simulink model "distributed"  (R2022a)
settings: Solver=VariableStepAuto  StartTime=0.0  StopTime=T_fin  FixedStep=0.0025  RelTol=1e-3
values from neighbouring files (symbols this model uses):
  A = A-B*k_leader    [project.m]
  Ad = [0 0 1 0 0 0; 1 0 0 0 0 0;0 1 0 0 0 0; 1 0 0 0 0 0; 0 0 0 0 0 0; 0 0 1 0 0 0]    [project.m]
  B = [0; -9.9453]    [project.m]
  C = [708.27 0]    [project.m]
  c = 5    [project.m]
  D_ = zeros(2,1)'    [project.m]
  F = P2*C'*inv(R)    [project.m]
  G = diag([1 0 0 0 1 0])    [project.m]
  K = inv(R)*B'*P    [project.m]
  L_leader = acker(A',C',[-1,-2])'    [project.m]
  X0 = [1/C(1) 1/800]'    [project.m]
settings Model: Creator=Giacomo  LastModifiedBy=Utente
settings DataIOCC: ReturnWorkspaceOutputs=off

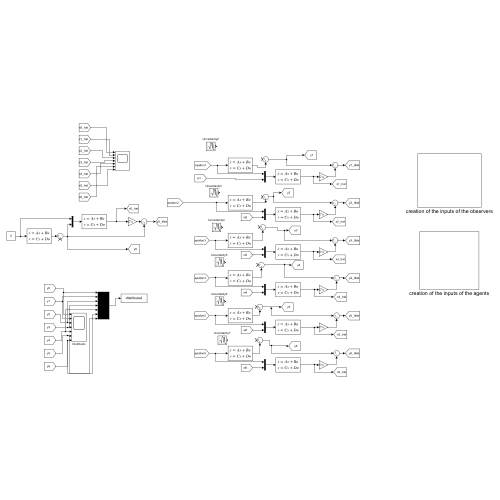
[thumbnail: Simulink's stored preview of the top-level diagram]
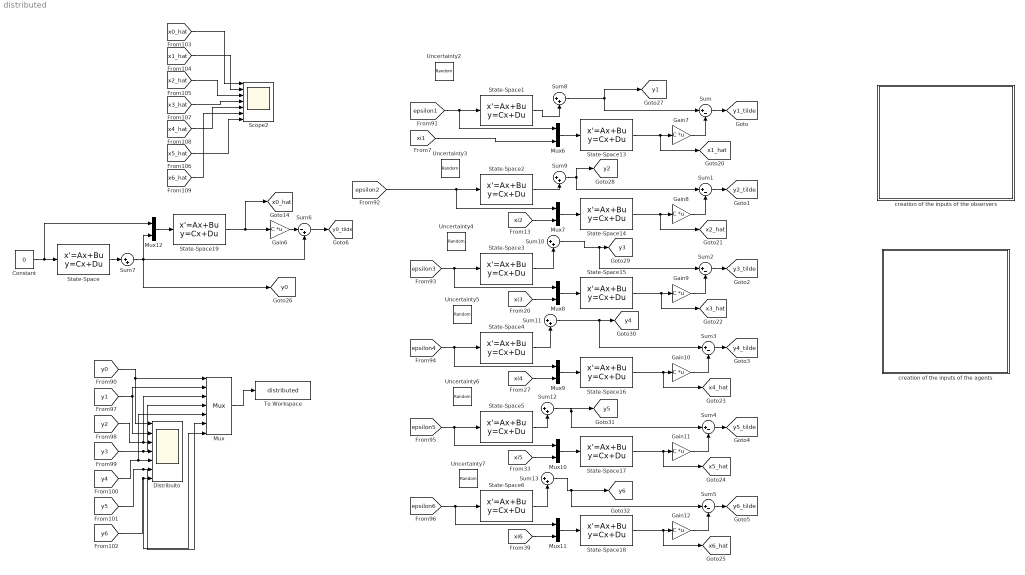
== system distributed ==
  Constant : Constant  Value=0
  Distribuito : Scope  NumInputPorts=7
  Gain{6..12} (7 alike) : Gain  Gain=C  Multiplication=Matrix(K*u)
  Mux : Mux  Inputs=7
  Mux{6..12} (7 alike) : Mux  Inputs=2
  Scope2 : Scope  NumInputPorts=7
  State-Space : StateSpace  A=A  B=B  C=C  D=0  InitialCondition=X0
  State-Space1 : StateSpace  A=A  B=B*c*K  C=C  D=D_  InitialCondition=[2/C(1) 1/800]'
  State-Space{13..18} (6 alike) : StateSpace  A=A  B=[B*c*K -c*F]  C=eye(2)  D=zeros(2,3)  InitialCondition=zeros(1,2)
  State-Space19 : StateSpace  A=A - L_leader*C  B=[B L_leader]  C=eye(2)  D=zeros(2,2)  InitialCondition=zeros(1,2)
  State-Space2 : StateSpace  A=A  B=B*c*K  C=C  D=D_  InitialCondition=[0 2/800]'
  State-Space3 : StateSpace  A=A  B=B*c*K  C=C  D=D_  InitialCondition=[-1/C(1) -1/800]
  State-Space4 : StateSpace  A=A  B=B*c*K  C=C  D=D_  InitialCondition=[3/C(1) -3/800]'
  State-Space5 : StateSpace  A=A  B=B*c*K  C=C  D=D_  InitialCondition=[2/C(1) 4/800]'
  State-Space6 : StateSpace  A=A  B=B*c*K  C=C  D=D_  InitialCondition=[-2/C(1) 0]'
  Sum{,1..5} (6 alike) : Sum  Inputs=|+-
  Sum{7..13} (7 alike) : Sum  Inputs=|++
  Sum6 : Sum  Inputs=|-+
  To Workspace : ToWorkspace  VariableName=distributed  SaveFormat=Timeseries  SampleTime=-1
  Uncertainty2 : RandomNumber  Mean=zeros(1,1)  Seed=2  SampleTime=0.2
  Uncertainty3 : RandomNumber  Mean=zeros(1,1)  Variance=0.5  Seed=7  SampleTime=0.1
  Uncertainty4 : RandomNumber  Mean=zeros(1,1)  Variance=0.2  Seed=7  SampleTime=0.1
  Uncertainty5 : RandomNumber  Mean=zeros(1,1)  Variance=0.7  Seed=3  SampleTime=0.1
  Uncertainty6 : RandomNumber  Mean=zeros(1,1)  Variance=0.1  Seed=1  SampleTime=0.1
  Uncertainty7 : RandomNumber  Mean=zeros(1,1)  Variance=0.4  Seed=3  SampleTime=0.1
  creation of the inputs of the agents : Subsystem
  creation of the inputs of the observers : Subsystem
  tag scope: x0_hat=global, x1_hat=global, x2_hat=global, x3_hat=global, x4_hat=global, x5_hat=global, x6_hat=global, y0=global, y0_tilde=global, y1=global, y1_tilde=global, y2=global, y2_tilde=global, y3=global, y3_tilde=global, y4=global, y4_tilde=global, y5=global, y5_tilde=global, y6=global, y6_tilde=global
  wires:
  Gain7/1 -> Sum/2
  Sum2/1 -> [y3_tilde]
  [xi2] -> Mux7/2
  [xi6] -> Mux11/2
  Mux8/1 -> State-Space15/1
  [xi3] -> Mux8/2
  [xi4] -> Mux9/2
  [xi5] -> Mux10/2
  [epsilon3] -> Mux8/1, State-Space3/1
  Mux6/1 -> State-Space13/1
  [epsilon6] -> State-Space6/1, Mux11/1
  [epsilon1] -> Mux6/1, State-Space1/1
  [epsilon5] -> State-Space5/1, Mux10/1
  Mux12/1 -> State-Space19/1
  Sum4/1 -> [y5_tilde]
  Mux9/1 -> State-Space16/1
  Sum5/1 -> [y6_tilde]
  Sum1/1 -> [y2_tilde]
  Gain12/1 -> Sum5/2
  [xi1] -> Mux6/2
  State-Space14/1 -> [x2_hat], Gain8/1
  [epsilon2] -> State-Space2/1, Mux7/1
  State-Space13/1 -> Gain7/1, [x1_hat]
  State-Space17/1 -> [x5_hat], Gain11/1
  Sum/1 -> [y1_tilde]
  Sum3/1 -> [y4_tilde]
  Gain11/1 -> Sum4/2
  State-Space19/1 -> Gain6/1, [x0_hat]
  [epsilon4] -> State-Space4/1, Mux9/1
  State-Space18/1 -> [x6_hat], Gain12/1
  State-Space15/1 -> [x3_hat], Gain9/1
  Gain8/1 -> Sum1/2
  Mux11/1 -> State-Space18/1
  Gain10/1 -> Sum3/2
  Sum6/1 -> [y0_tilde]
  State-Space16/1 -> [x4_hat], Gain10/1
  Gain9/1 -> Sum2/2
  Mux10/1 -> State-Space17/1
  Constant/1 -> Mux12/1, State-Space/1
  [y6] -> Mux/7, Distribuito/7
  [y5] -> Mux/6, Distribuito/6
  [y4] -> Distribuito/5, Mux/5
  [y3] -> Mux/4, Distribuito/4
  [y2] -> Mux/3, Distribuito/3
  [y1] -> Mux/2, Distribuito/2
  [y0] -> Mux/1, Distribuito/1
  Gain6/1 -> Sum6/1
  State-Space/1 -> Sum7/1
  Sum7/1 -> Mux12/2, Sum6/2, [y0]
  State-Space1/1 -> Sum8/2
  Sum8/1 -> [y1], Sum/1
  State-Space2/1 -> Sum9/2
  Sum9/1 -> Sum1/1, [y2]
  State-Space3/1 -> Sum10/2
  Sum10/1 -> Sum2/1, [y3]
  State-Space4/1 -> Sum11/2
  Sum11/1 -> Sum3/1, [y4]
  State-Space5/1 -> Sum12/2
  Sum12/1 -> Sum4/1, [y5]
  State-Space6/1 -> Sum13/2
  Sum13/1 -> Sum5/1, [y6]
  Mux/1 -> To Workspace/1
  [x0_hat] -> Scope2/1
  [x6_hat] -> Scope2/6
  [x3_hat] -> Scope2/4
  [x1_hat] -> Scope2/2
  [x2_hat] -> Scope2/3
  [x4_hat] -> Scope2/5
  [x5_hat] -> Scope2/7
  Mux7/1 -> State-Space14/1

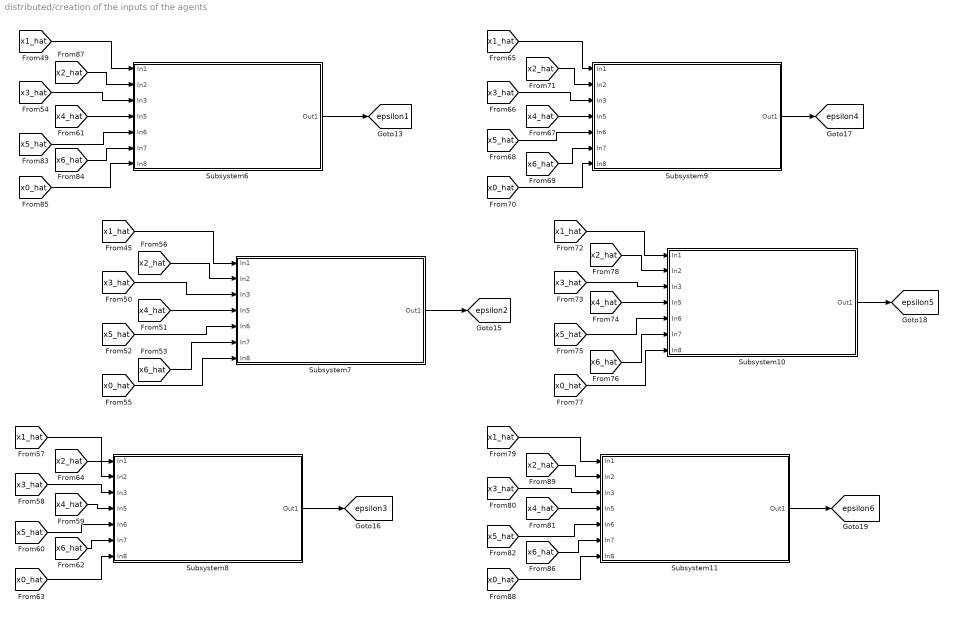
== system distributed/creation of the inputs of the agents ==
  Subsystem10 : Subsystem
  Subsystem11 : Subsystem
  Subsystem6 : Subsystem
  Subsystem7 : Subsystem
  Subsystem8 : Subsystem
  Subsystem9 : Subsystem
  tag scope: epsilon1=global, epsilon2=global, epsilon3=global, epsilon4=global, epsilon5=global, epsilon6=global
  wires:
  [x2_hat] -> Subsystem11/2(In2)
  Subsystem7/1(Out1) -> [epsilon2]
  [x1_hat] -> Subsystem10/1(In1)
  [x6_hat] -> Subsystem6/6(In7)
  [x3_hat] -> Subsystem8/3(In3)
  [x3_hat] -> Subsystem11/3(In3)
  [x5_hat] -> Subsystem6/5(In6)
  [x6_hat] -> Subsystem11/6(In7)
  [x4_hat] -> Subsystem6/4(In5)
  [x0_hat] -> Subsystem7/7(In8)
  [x1_hat] -> Subsystem9/1(In1)
  [x5_hat] -> Subsystem11/5(In6)
  Subsystem11/1(Out1) -> [epsilon6]
  [x3_hat] -> Subsystem10/3(In3)
  [x4_hat] -> Subsystem8/4(In5)
  Subsystem10/1(Out1) -> [epsilon5]
  [x3_hat] -> Subsystem7/3(In3)
  [x3_hat] -> Subsystem9/3(In3)
  Subsystem9/1(Out1) -> [epsilon4]
  [x0_hat] -> Subsystem10/7(In8)
  [x1_hat] -> Subsystem8/1(In1)
  [x6_hat] -> Subsystem7/6(In7)
  [x0_hat] -> Subsystem8/7(In8)
  [x5_hat] -> Subsystem10/5(In6)
  [x6_hat] -> Subsystem10/6(In7)
  [x5_hat] -> Subsystem7/5(In6)
  [x2_hat] -> Subsystem10/2(In2)
  [x4_hat] -> Subsystem7/4(In5)
  [x0_hat] -> Subsystem9/7(In8)
  [x4_hat] -> Subsystem9/4(In5)
  [x2_hat] -> Subsystem9/2(In2)
  Subsystem8/1(Out1) -> [epsilon3]
  [x5_hat] -> Subsystem8/5(In6)
  [x5_hat] -> Subsystem9/5(In6)
  [x4_hat] -> Subsystem10/4(In5)
  [x4_hat] -> Subsystem11/4(In5)
  [x1_hat] -> Subsystem7/1(In1)
  [x3_hat] -> Subsystem6/3(In3)
  [x0_hat] -> Subsystem11/7(In8)
  [x2_hat] -> Subsystem7/2(In2)
  Subsystem6/1(Out1) -> [epsilon1]
  [x0_hat] -> Subsystem6/7(In8)
  [x1_hat] -> Subsystem11/1(In1)
  [x2_hat] -> Subsystem8/2(In2)
  [x6_hat] -> Subsystem9/6(In7)
  [x2_hat] -> Subsystem6/2(In2)
  [x1_hat] -> Subsystem6/1(In1)
  [x6_hat] -> Subsystem8/6(In7)

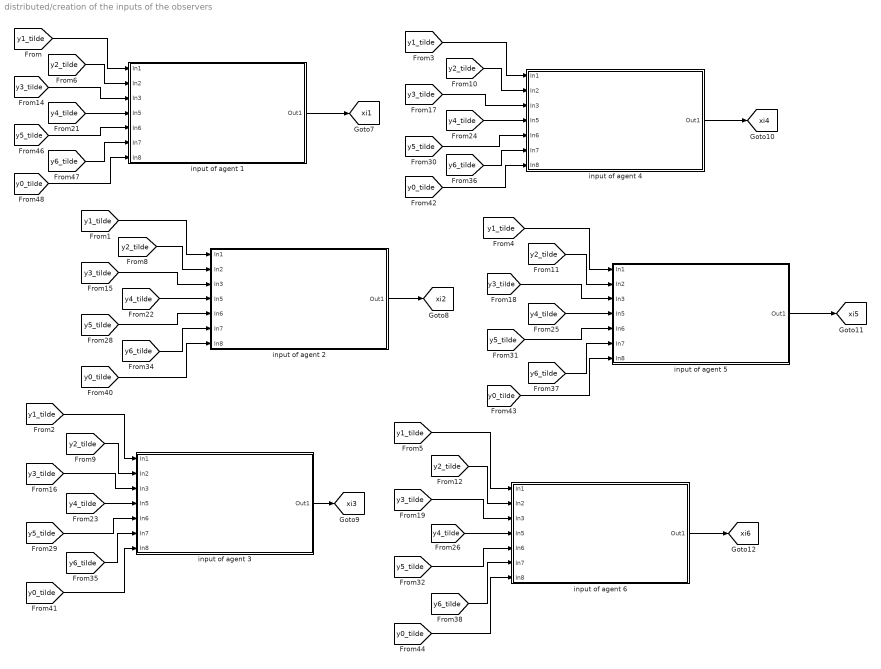
== system distributed/creation of the inputs of the observers ==
  input of agent 1 : Subsystem
  input of agent 2 : Subsystem
  input of agent 3 : Subsystem
  input of agent 4 : Subsystem
  input of agent 5 : Subsystem
  input of agent 6 : Subsystem
  tag scope: xi1=global, xi2=global, xi3=global, xi4=global, xi5=global, xi6=global
  wires:
  [y6_tilde] -> input of agent 5/6(In7)
  [y2_tilde] -> input of agent 2/2(In2)
  [y5_tilde] -> input of agent 3/5(In6)
  [y2_tilde] -> input of agent 5/2(In2)
  [y0_tilde] -> input of agent 1/7(In8)
  [y5_tilde] -> input of agent 4/5(In6)
  [y6_tilde] -> input of agent 4/6(In7)
  [y0_tilde] -> input of agent 6/7(In8)
  [y5_tilde] -> input of agent 1/5(In6)
  input of agent 3/1(Out1) -> [xi3]
  [y1_tilde] -> input of agent 3/1(In1)
  [y0_tilde] -> input of agent 3/7(In8)
  [y1_tilde] -> input of agent 2/1(In1)
  [y5_tilde] -> input of agent 5/5(In6)
  input of agent 6/1(Out1) -> [xi6]
  [y6_tilde] -> input of agent 3/6(In7)
  [y4_tilde] -> input of agent 4/4(In5)
  [y3_tilde] -> input of agent 4/3(In3)
  [y6_tilde] -> input of agent 1/6(In7)
  [y1_tilde] -> input of agent 1/1(In1)
  [y4_tilde] -> input of agent 1/4(In5)
  [y2_tilde] -> input of agent 6/2(In2)
  [y2_tilde] -> input of agent 4/2(In2)
  [y3_tilde] -> input of agent 3/3(In3)
  [y5_tilde] -> input of agent 6/5(In6)
  [y6_tilde] -> input of agent 2/6(In7)
  [y4_tilde] -> input of agent 5/4(In5)
  [y3_tilde] -> input of agent 5/3(In3)
  [y4_tilde] -> input of agent 6/4(In5)
  [y0_tilde] -> input of agent 4/7(In8)
  [y0_tilde] -> input of agent 5/7(In8)
  [y1_tilde] -> input of agent 6/1(In1)
  [y4_tilde] -> input of agent 2/4(In5)
  input of agent 1/1(Out1) -> [xi1]
  [y3_tilde] -> input of agent 6/3(In3)
  [y3_tilde] -> input of agent 1/3(In3)
  [y6_tilde] -> input of agent 6/6(In7)
  [y1_tilde] -> input of agent 4/1(In1)
  [y3_tilde] -> input of agent 2/3(In3)
  [y4_tilde] -> input of agent 3/4(In5)
  [y2_tilde] -> input of agent 3/2(In2)
  [y0_tilde] -> input of agent 2/7(In8)
  input of agent 4/1(Out1) -> [xi4]
  input of agent 2/1(Out1) -> [xi2]
  [y5_tilde] -> input of agent 2/5(In6)
  [y1_tilde] -> input of agent 5/1(In1)
  [y2_tilde] -> input of agent 1/2(In2)
  input of agent 5/1(Out1) -> [xi5]

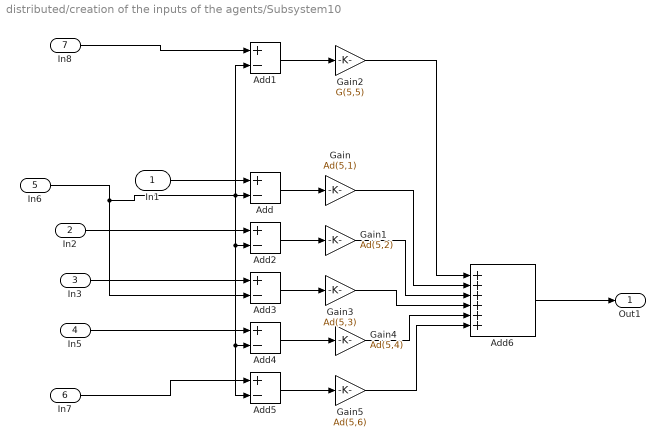
== system distributed/creation of the inputs of the agents/Subsystem10 ==
  In1 : Inport
  In2 : Inport  Port=2
  In3 : Inport  Port=3
  In5 : Inport  Port=4
  In6 : Inport  Port=5
  In7 : Inport  Port=6
  In8 : Inport  Port=7
  Add{,1..5} (6 alike) : Sum  Inputs=+-
  Add6 : Sum  Inputs=++++++
  Gain : Gain  Gain=Ad(5,1)
  Gain1 : Gain  Gain=Ad(5,2)
  Gain2 : Gain  Gain=G(5,5)
  Gain3 : Gain  Gain=Ad(5,3)
  Gain4 : Gain  Gain=Ad(5,4)
  Gain5 : Gain  Gain=Ad(5,6)
  Out1 : Outport
  wires:
  Add/1 -> Gain/1
  In6/1 -> Add3/2, Add5/2, Add4/2, Add2/2, Add/2, Add1/2
  In8/1 -> Add1/1
  Add2/1 -> Gain1/1
  Add3/1 -> Gain3/1
  Add4/1 -> Gain4/1
  Add5/1 -> Gain5/1
  In2/1 -> Add2/1
  In3/1 -> Add3/1
  In5/1 -> Add4/1
  In7/1 -> Add5/1
  Gain/1 -> Add6/2
  Gain1/1 -> Add6/3
  Gain3/1 -> Add6/4
  Gain4/1 -> Add6/5
  Gain5/1 -> Add6/6
  Add1/1 -> Gain2/1
  Gain2/1 -> Add6/1
  Add6/1 -> Out1/1
  In1/1 -> Add/1

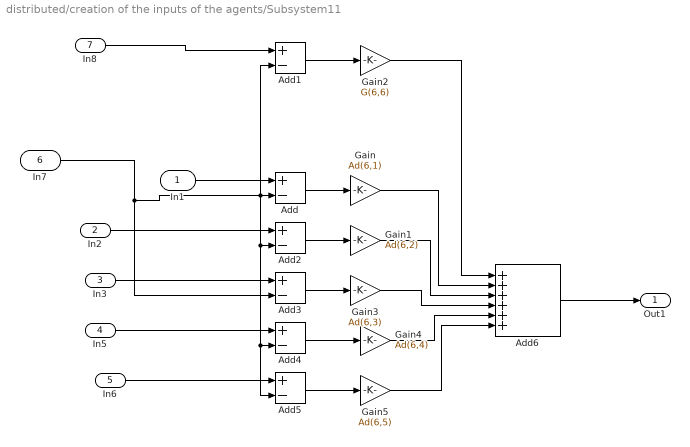
== system distributed/creation of the inputs of the agents/Subsystem11 ==
  In1 : Inport
  In2 : Inport  Port=2
  In3 : Inport  Port=3
  In5 : Inport  Port=4
  In6 : Inport  Port=5
  In7 : Inport  Port=6
  In8 : Inport  Port=7
  Add{,1..5} (6 alike) : Sum  Inputs=+-
  Add6 : Sum  Inputs=++++++
  Gain : Gain  Gain=Ad(6,1)
  Gain1 : Gain  Gain=Ad(6,2)
  Gain2 : Gain  Gain=G(6,6)
  Gain3 : Gain  Gain=Ad(6,3)
  Gain4 : Gain  Gain=Ad(6,4)
  Gain5 : Gain  Gain=Ad(6,5)
  Out1 : Outport
  wires:
  Add/1 -> Gain/1
  In7/1 -> Add3/2, Add5/2, Add4/2, Add2/2, Add/2, Add1/2
  In8/1 -> Add1/1
  Add2/1 -> Gain1/1
  Add3/1 -> Gain3/1
  Add4/1 -> Gain4/1
  Add5/1 -> Gain5/1
  In2/1 -> Add2/1
  In3/1 -> Add3/1
  In5/1 -> Add4/1
  In6/1 -> Add5/1
  Gain/1 -> Add6/2
  Gain1/1 -> Add6/3
  Gain3/1 -> Add6/4
  Gain4/1 -> Add6/5
  Gain5/1 -> Add6/6
  Add1/1 -> Gain2/1
  Gain2/1 -> Add6/1
  Add6/1 -> Out1/1
  In1/1 -> Add/1

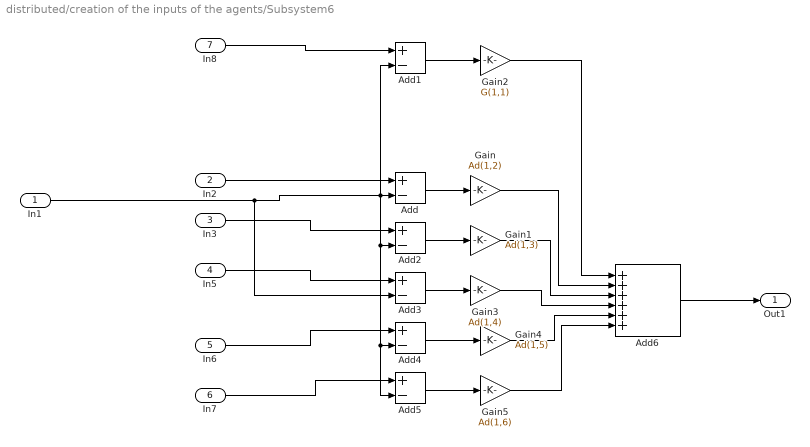
== system distributed/creation of the inputs of the agents/Subsystem6 ==
  In1 : Inport
  In2 : Inport  Port=2
  In3 : Inport  Port=3
  In5 : Inport  Port=4
  In6 : Inport  Port=5
  In7 : Inport  Port=6
  In8 : Inport  Port=7
  Add{,1..5} (6 alike) : Sum  Inputs=+-
  Add6 : Sum  Inputs=++++++
  Gain : Gain  Gain=Ad(1,2)
  Gain1 : Gain  Gain=Ad(1,3)
  Gain2 : Gain  Gain=G(1,1)
  Gain3 : Gain  Gain=Ad(1,4)
  Gain4 : Gain  Gain=Ad(1,5)
  Gain5 : Gain  Gain=Ad(1,6)
  Out1 : Outport
  wires:
  Add/1 -> Gain/1
  In1/1 -> Add3/2, Add5/2, Add4/2, Add2/2, Add/2, Add1/2
  In2/1 -> Add/1
  In8/1 -> Add1/1
  Add2/1 -> Gain1/1
  Add3/1 -> Gain3/1
  Add4/1 -> Gain4/1
  Add5/1 -> Gain5/1
  In3/1 -> Add2/1
  In5/1 -> Add3/1
  In6/1 -> Add4/1
  In7/1 -> Add5/1
  Gain/1 -> Add6/2
  Gain1/1 -> Add6/3
  Gain3/1 -> Add6/4
  Gain4/1 -> Add6/5
  Gain5/1 -> Add6/6
  Add1/1 -> Gain2/1
  Gain2/1 -> Add6/1
  Add6/1 -> Out1/1

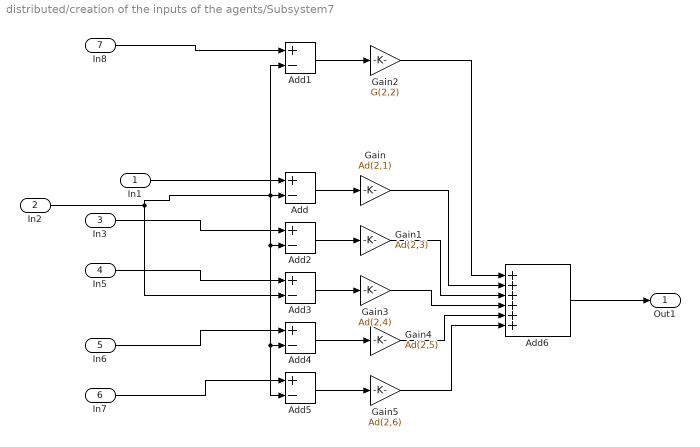
== system distributed/creation of the inputs of the agents/Subsystem7 ==
  In1 : Inport
  In2 : Inport  Port=2
  In3 : Inport  Port=3
  In5 : Inport  Port=4
  In6 : Inport  Port=5
  In7 : Inport  Port=6
  In8 : Inport  Port=7
  Add{,1..5} (6 alike) : Sum  Inputs=+-
  Add6 : Sum  Inputs=++++++
  Gain : Gain  Gain=Ad(2,1)
  Gain1 : Gain  Gain=Ad(2,3)
  Gain2 : Gain  Gain=G(2,2)
  Gain3 : Gain  Gain=Ad(2,4)
  Gain4 : Gain  Gain=Ad(2,5)
  Gain5 : Gain  Gain=Ad(2,6)
  Out1 : Outport
  wires:
  Add/1 -> Gain/1
  In2/1 -> Add3/2, Add5/2, Add4/2, Add2/2, Add/2, Add1/2
  In1/1 -> Add/1
  In8/1 -> Add1/1
  Add2/1 -> Gain1/1
  Add3/1 -> Gain3/1
  Add4/1 -> Gain4/1
  Add5/1 -> Gain5/1
  In3/1 -> Add2/1
  In5/1 -> Add3/1
  In6/1 -> Add4/1
  In7/1 -> Add5/1
  Gain/1 -> Add6/2
  Gain1/1 -> Add6/3
  Gain3/1 -> Add6/4
  Gain4/1 -> Add6/5
  Gain5/1 -> Add6/6
  Add1/1 -> Gain2/1
  Gain2/1 -> Add6/1
  Add6/1 -> Out1/1

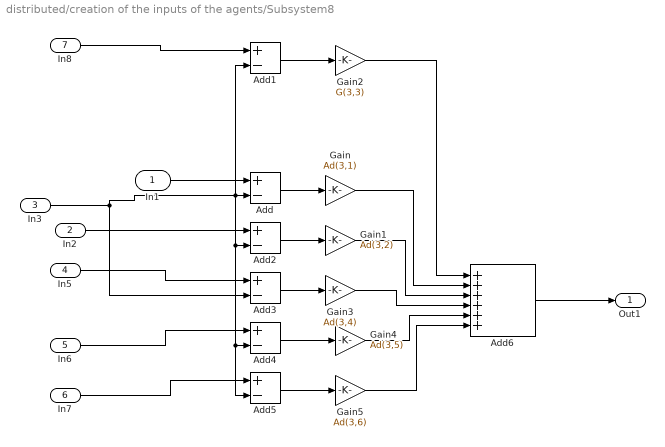
== system distributed/creation of the inputs of the agents/Subsystem8 ==
  In1 : Inport
  In2 : Inport  Port=2
  In3 : Inport  Port=3
  In5 : Inport  Port=4
  In6 : Inport  Port=5
  In7 : Inport  Port=6
  In8 : Inport  Port=7
  Add{,1..5} (6 alike) : Sum  Inputs=+-
  Add6 : Sum  Inputs=++++++
  Gain : Gain  Gain=Ad(3,1)
  Gain1 : Gain  Gain=Ad(3,2)
  Gain2 : Gain  Gain=G(3,3)
  Gain3 : Gain  Gain=Ad(3,4)
  Gain4 : Gain  Gain=Ad(3,5)
  Gain5 : Gain  Gain=Ad(3,6)
  Out1 : Outport
  wires:
  Add/1 -> Gain/1
  In3/1 -> Add3/2, Add5/2, Add4/2, Add2/2, Add/2, Add1/2
  In8/1 -> Add1/1
  Add2/1 -> Gain1/1
  Add3/1 -> Gain3/1
  Add4/1 -> Gain4/1
  Add5/1 -> Gain5/1
  In2/1 -> Add2/1
  In5/1 -> Add3/1
  In6/1 -> Add4/1
  In7/1 -> Add5/1
  Gain/1 -> Add6/2
  Gain1/1 -> Add6/3
  Gain3/1 -> Add6/4
  Gain4/1 -> Add6/5
  Gain5/1 -> Add6/6
  Add1/1 -> Gain2/1
  Gain2/1 -> Add6/1
  Add6/1 -> Out1/1
  In1/1 -> Add/1

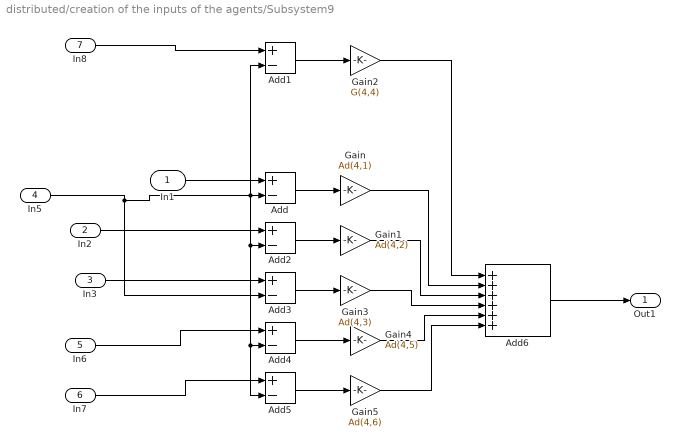
== system distributed/creation of the inputs of the agents/Subsystem9 ==
  In1 : Inport
  In2 : Inport  Port=2
  In3 : Inport  Port=3
  In5 : Inport  Port=4
  In6 : Inport  Port=5
  In7 : Inport  Port=6
  In8 : Inport  Port=7
  Add{,1..5} (6 alike) : Sum  Inputs=+-
  Add6 : Sum  Inputs=++++++
  Gain : Gain  Gain=Ad(4,1)
  Gain1 : Gain  Gain=Ad(4,2)
  Gain2 : Gain  Gain=G(4,4)
  Gain3 : Gain  Gain=Ad(4,3)
  Gain4 : Gain  Gain=Ad(4,5)
  Gain5 : Gain  Gain=Ad(4,6)
  Out1 : Outport
  wires:
  Add/1 -> Gain/1
  In5/1 -> Add3/2, Add5/2, Add4/2, Add2/2, Add/2, Add1/2
  In8/1 -> Add1/1
  Add2/1 -> Gain1/1
  Add3/1 -> Gain3/1
  Add4/1 -> Gain4/1
  Add5/1 -> Gain5/1
  In2/1 -> Add2/1
  In3/1 -> Add3/1
  In6/1 -> Add4/1
  In7/1 -> Add5/1
  Gain/1 -> Add6/2
  Gain1/1 -> Add6/3
  Gain3/1 -> Add6/4
  Gain4/1 -> Add6/5
  Gain5/1 -> Add6/6
  Add1/1 -> Gain2/1
  Gain2/1 -> Add6/1
  Add6/1 -> Out1/1
  In1/1 -> Add/1

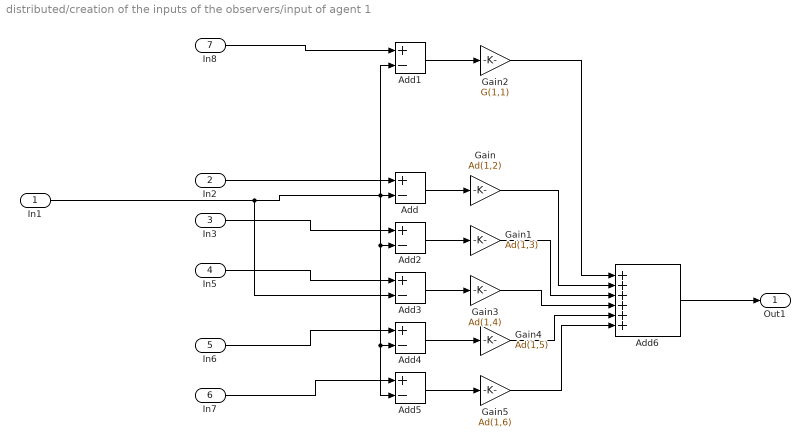
== system distributed/creation of the inputs of the observers/input of agent 1 ==
  In1 : Inport
  In2 : Inport  Port=2
  In3 : Inport  Port=3
  In5 : Inport  Port=4
  In6 : Inport  Port=5
  In7 : Inport  Port=6
  In8 : Inport  Port=7
  Add{,1..5} (6 alike) : Sum  Inputs=+-
  Add6 : Sum  Inputs=++++++
  Gain : Gain  Gain=Ad(1,2)
  Gain1 : Gain  Gain=Ad(1,3)
  Gain2 : Gain  Gain=G(1,1)
  Gain3 : Gain  Gain=Ad(1,4)
  Gain4 : Gain  Gain=Ad(1,5)
  Gain5 : Gain  Gain=Ad(1,6)
  Out1 : Outport
  wires:
  Add/1 -> Gain/1
  In1/1 -> Add3/2, Add5/2, Add4/2, Add2/2, Add/2, Add1/2
  In2/1 -> Add/1
  In8/1 -> Add1/1
  Add2/1 -> Gain1/1
  Add3/1 -> Gain3/1
  Add4/1 -> Gain4/1
  Add5/1 -> Gain5/1
  In3/1 -> Add2/1
  In5/1 -> Add3/1
  In6/1 -> Add4/1
  In7/1 -> Add5/1
  Gain/1 -> Add6/2
  Gain1/1 -> Add6/3
  Gain3/1 -> Add6/4
  Gain4/1 -> Add6/5
  Gain5/1 -> Add6/6
  Add1/1 -> Gain2/1
  Gain2/1 -> Add6/1
  Add6/1 -> Out1/1

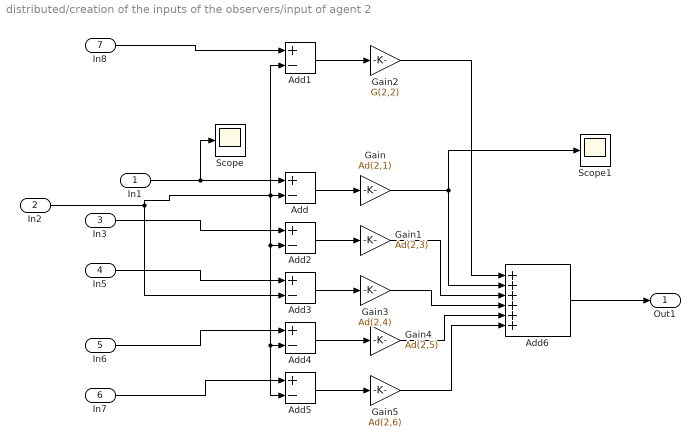
== system distributed/creation of the inputs of the observers/input of agent 2 ==
  In1 : Inport
  In2 : Inport  Port=2
  In3 : Inport  Port=3
  In5 : Inport  Port=4
  In6 : Inport  Port=5
  In7 : Inport  Port=6
  In8 : Inport  Port=7
  Add{,1..5} (6 alike) : Sum  Inputs=+-
  Add6 : Sum  Inputs=++++++
  Gain : Gain  Gain=Ad(2,1)
  Gain1 : Gain  Gain=Ad(2,3)
  Gain2 : Gain  Gain=G(2,2)
  Gain3 : Gain  Gain=Ad(2,4)
  Gain4 : Gain  Gain=Ad(2,5)
  Gain5 : Gain  Gain=Ad(2,6)
  Scope : Scope
  Scope1 : Scope
  Out1 : Outport
  wires:
  Add/1 -> Gain/1
  In2/1 -> Add3/2, Add5/2, Add4/2, Add2/2, Add/2, Add1/2
  In1/1 -> Scope/1, Add/1
  In8/1 -> Add1/1
  Add2/1 -> Gain1/1
  Add3/1 -> Gain3/1
  Add4/1 -> Gain4/1
  Add5/1 -> Gain5/1
  In3/1 -> Add2/1
  In5/1 -> Add3/1
  In6/1 -> Add4/1
  In7/1 -> Add5/1
  Gain/1 -> Scope1/1, Add6/2
  Gain1/1 -> Add6/3
  Gain3/1 -> Add6/4
  Gain4/1 -> Add6/5
  Gain5/1 -> Add6/6
  Add1/1 -> Gain2/1
  Gain2/1 -> Add6/1
  Add6/1 -> Out1/1

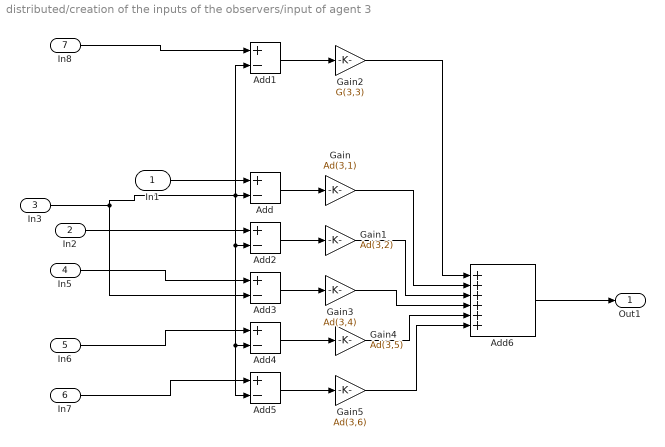
== system distributed/creation of the inputs of the observers/input of agent 3 ==
  In1 : Inport
  In2 : Inport  Port=2
  In3 : Inport  Port=3
  In5 : Inport  Port=4
  In6 : Inport  Port=5
  In7 : Inport  Port=6
  In8 : Inport  Port=7
  Add{,1..5} (6 alike) : Sum  Inputs=+-
  Add6 : Sum  Inputs=++++++
  Gain : Gain  Gain=Ad(3,1)
  Gain1 : Gain  Gain=Ad(3,2)
  Gain2 : Gain  Gain=G(3,3)
  Gain3 : Gain  Gain=Ad(3,4)
  Gain4 : Gain  Gain=Ad(3,5)
  Gain5 : Gain  Gain=Ad(3,6)
  Out1 : Outport
  wires:
  Add/1 -> Gain/1
  In3/1 -> Add3/2, Add1/2, Add5/2, Add4/2, Add2/2, Add/2
  In8/1 -> Add1/1
  Add2/1 -> Gain1/1
  Add3/1 -> Gain3/1
  Add4/1 -> Gain4/1
  Add5/1 -> Gain5/1
  In2/1 -> Add2/1
  In5/1 -> Add3/1
  In6/1 -> Add4/1
  In7/1 -> Add5/1
  Gain/1 -> Add6/2
  Gain1/1 -> Add6/3
  Gain3/1 -> Add6/4
  Gain4/1 -> Add6/5
  Gain5/1 -> Add6/6
  Add1/1 -> Gain2/1
  Gain2/1 -> Add6/1
  Add6/1 -> Out1/1
  In1/1 -> Add/1

== system distributed/creation of the inputs of the observers/input of agent 4 ==
  In1 : Inport
  In2 : Inport  Port=2
  In3 : Inport  Port=3
  In5 : Inport  Port=4
  In6 : Inport  Port=5
  In7 : Inport  Port=6
  In8 : Inport  Port=7
  Add{,1..5} (6 alike) : Sum  Inputs=+-
  Add6 : Sum  Inputs=++++++
  Gain : Gain  Gain=Ad(4,1)
  Gain1 : Gain  Gain=Ad(4,2)
  Gain2 : Gain  Gain=G(4,4)
  Gain3 : Gain  Gain=Ad(4,3)
  Gain4 : Gain  Gain=Ad(4,5)
  Gain5 : Gain  Gain=Ad(4,6)
  Out1 : Outport
  wires:
  Add/1 -> Gain/1
  In5/1 -> Add3/2, Add5/2, Add4/2, Add2/2, Add/2, Add1/2
  In8/1 -> Add1/1
  Add2/1 -> Gain1/1
  Add3/1 -> Gain3/1
  Add4/1 -> Gain4/1
  Add5/1 -> Gain5/1
  In2/1 -> Add2/1
  In3/1 -> Add3/1
  In6/1 -> Add4/1
  In7/1 -> Add5/1
  Gain/1 -> Add6/2
  Gain1/1 -> Add6/3
  Gain3/1 -> Add6/4
  Gain4/1 -> Add6/5
  Gain5/1 -> Add6/6
  Add1/1 -> Gain2/1
  Gain2/1 -> Add6/1
  Add6/1 -> Out1/1
  In1/1 -> Add/1

== system distributed/creation of the inputs of the observers/input of agent 5 ==
  In1 : Inport
  In2 : Inport  Port=2
  In3 : Inport  Port=3
  In5 : Inport  Port=4
  In6 : Inport  Port=5
  In7 : Inport  Port=6
  In8 : Inport  Port=7
  Add{,1..5} (6 alike) : Sum  Inputs=+-
  Add6 : Sum  Inputs=++++++
  Gain : Gain  Gain=Ad(5,1)
  Gain1 : Gain  Gain=Ad(5,2)
  Gain2 : Gain  Gain=G(5,5)
  Gain3 : Gain  Gain=Ad(5,3)
  Gain4 : Gain  Gain=Ad(5,4)
  Gain5 : Gain  Gain=Ad(5,6)
  Out1 : Outport
  wires:
  Add/1 -> Gain/1
  In6/1 -> Add3/2, Add5/2, Add4/2, Add2/2, Add/2, Add1/2
  In8/1 -> Add1/1
  Add2/1 -> Gain1/1
  Add3/1 -> Gain3/1
  Add4/1 -> Gain4/1
  Add5/1 -> Gain5/1
  In2/1 -> Add2/1
  In3/1 -> Add3/1
  In5/1 -> Add4/1
  In7/1 -> Add5/1
  Gain/1 -> Add6/2
  Gain1/1 -> Add6/3
  Gain3/1 -> Add6/4
  Gain4/1 -> Add6/5
  Gain5/1 -> Add6/6
  Add1/1 -> Gain2/1
  Gain2/1 -> Add6/1
  Add6/1 -> Out1/1
  In1/1 -> Add/1

== system distributed/creation of the inputs of the observers/input of agent 6 ==
  In1 : Inport
  In2 : Inport  Port=2
  In3 : Inport  Port=3
  In5 : Inport  Port=4
  In6 : Inport  Port=5
  In7 : Inport  Port=6
  In8 : Inport  Port=7
  Add{,1..5} (6 alike) : Sum  Inputs=+-
  Add6 : Sum  Inputs=++++++
  Gain : Gain  Gain=Ad(6,1)
  Gain1 : Gain  Gain=Ad(6,2)
  Gain2 : Gain  Gain=G(6,6)
  Gain3 : Gain  Gain=Ad(6,3)
  Gain4 : Gain  Gain=Ad(6,4)
  Gain5 : Gain  Gain=Ad(6,5)
  Out1 : Outport
  wires:
  Add/1 -> Gain/1
  In7/1 -> Add3/2, Add5/2, Add4/2, Add2/2, Add/2, Add1/2
  In8/1 -> Add1/1
  Add2/1 -> Gain1/1
  Add3/1 -> Gain3/1
  Add4/1 -> Gain4/1
  Add5/1 -> Gain5/1
  In2/1 -> Add2/1
  In3/1 -> Add3/1
  In5/1 -> Add4/1
  In6/1 -> Add5/1
  Gain/1 -> Add6/2
  Gain1/1 -> Add6/3
  Gain3/1 -> Add6/4
  Gain4/1 -> Add6/5
  Gain5/1 -> Add6/6
  Add1/1 -> Gain2/1
  Gain2/1 -> Add6/1
  Add6/1 -> Out1/1
  In1/1 -> Add/1
